simulink model "SA_Node_Ursino"  (Simulink 7.0)
settings: Solver=ode45  StartTime=0.0  StopTime=10.0  RelTol=1e-3
values from neighbouring files (symbols this model uses):
  ftbs_min = 0.1    [Cardiovascular_IC.m]    (also in SA_Node_Ursino_IC.m)
  HP_basal = 0.58    [Cardiovascular_IC.m]    (also in SA_Node_Ursino_IC.m)
undefined symbols (not defined in the file or in its folder): Dx, toux
settings Model: Creator=CLM  LastModifiedBy=CLM
settings DebuggingCC: SaveWithParameterizedLinksMsg=none  SignalResolutionControl=TryResolveAllWithWarning  MultiTaskDSMMsg=warning  MultiTaskCondExecSysMsg=none
settings RTWCC: IncludeERTFirstTime=on
settings GRTTargetCC: TargetFcnLib=ansi_tfl_tmw.mat

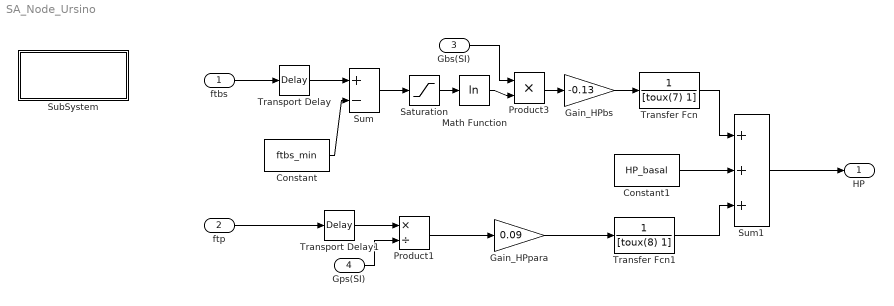
== system SA_Node_Ursino ==
  ftbs : Inport  OutDataType=sfix(16)  OutScaling=2^0
  ftp : Inport  Port=2  OutDataType=sfix(16)  OutScaling=2^0
  Gbs(SI) : Inport  Port=3  OutDataType=sfix(16)  OutScaling=2^0
  Gps(SI) : Inport  Port=4  OutDataType=sfix(16)  OutScaling=2^0
  Constant : Constant  Value=ftbs_min  OutDataType=sfix(16)  OutScaling=2^0
  Constant1 : Constant  Value=HP_basal  OutDataType=sfix(16)  OutScaling=2^0
  Gain_HPbs : Gain  Gain=-0.13  ParameterDataType=sfix(16)  ParameterScaling=2^0  OutDataType=sfix(16)  OutScaling=2^0  SaturateOnIntegerOverflow=on
  Gain_HPpara : Gain  Gain=0.09  ParameterDataType=sfix(16)  ParameterScaling=2^0  OutDataType=sfix(16)  OutScaling=2^0  SaturateOnIntegerOverflow=on
  Math Function : Math  Operator=log  OutDataType=sfix(16)  OutScaling=2^0  SaturateOnIntegerOverflow=on
  Product1 : Product  Inputs=*/  OutDataType=sfix(16)  OutScaling=2^0  SaturateOnIntegerOverflow=on  InputSameDT=on
  Product3 : Product  OutDataType=sfix(16)  OutScaling=2^0  SaturateOnIntegerOverflow=on  InputSameDT=on
  Saturation : Saturate  UpperLimit=inf  LowerLimit=1
  SubSystem : Subsystem
      settings: OpenFcn=pneuma_variables
      mask Display: disp('"double click here"\n to load SA Node \ninitial values');
  Sum : Sum  Inputs=+-  OutDataType=sfix(16)  OutScaling=2^0  SaturateOnIntegerOverflow=on  InputSameDT=on
  Sum1 : Sum  Inputs=+++  OutDataType=sfix(16)  OutScaling=2^0  SaturateOnIntegerOverflow=on  InputSameDT=on
  Transfer Fcn : TransferFcn  Denominator=[toux(7) 1]
  Transfer Fcn1 : TransferFcn  Denominator=[toux(8) 1]
  Transport Delay : TransportDelay  DelayTime=Dx(7)  BufferSize=19456
  Transport Delay1 : TransportDelay  DelayTime=Dx(8)  BufferSize=18432
  HP : Outport  OutDataType=sfix(16)  OutScaling=2^0
  wires:
  ftbs/1 -> Transport Delay/1
  Transport Delay/1 -> Sum/1
  Constant/1 -> Sum/2
  Sum/1 -> Saturation/1
  Saturation/1 -> Math Function/1
  Math Function/1 -> Product3/2
  Gain_HPbs/1 -> Transfer Fcn/1
  Transfer Fcn/1 -> Sum1/1
  Sum1/1 -> HP/1
  Constant1/1 -> Sum1/2
  ftp/1 -> Transport Delay1/1
  Transport Delay1/1 -> Product1/1
  Gain_HPpara/1 -> Transfer Fcn1/1
  Transfer Fcn1/1 -> Sum1/3
  Gbs(SI)/1 -> Product3/1
  Product3/1 -> Gain_HPbs/1
  Product1/1 -> Gain_HPpara/1
  Gps(SI)/1 -> Product1/2

== system SA_Node_Ursino/SubSystem ==
